simulink model "StateResetComponent"  (R2016a)
settings: Solver=ode45  StartTime=0.0  StopTime=10.0  RelTol=1e-3
settings Model: Creator=sz609516  LastModifiedBy=fhu
settings DataIOCC: LimitDataPoints=on  SaveFormat=Array
settings DebuggingCC: UnderspecifiedInitializationDetection=Classic  MergeDetectMultiDrivingBlocksExec=none  SolverPrmCheckMsg=warning  StateNameClashWarn=warning
settings HardwareCC: ProdBitPerPointer=32  ProdLargestAtomicFloat=None  ProdIntDivRoundTo=Undefined  ProdEndianess=Unspecified  ProdWordSize=32  ProdHWDeviceType=32-bit Generic
settings ModelReferenceCC: PropagateSignalLabelsOutOfModel=off
settings ConfigComp: CovModelRefEnable=Off

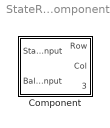
== system StateResetComponent ==
  Component : Subsystem

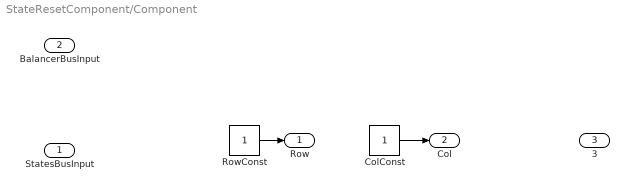
== system StateResetComponent/Component ==
  StatesBusInput : Inport
  BalancerBusInput : Inport  Port=2
  ColConst : Constant
  RowConst : Constant
  Row : Outport
  Col : Outport  Port=2
  3 : Outport  Port=3
  wires:
  RowConst/1 -> Row/1
  ColConst/1 -> Col/1
